simulink library "FadeControlBtc"  (R2022b)
settings: Solver=VariableStepAuto  StartTime=0.0  StopTime=10.0  RelTol=1e-3
undefined symbols (not defined in the file or in its folder): Row
libraries: TuneVar x6, TOP x2, FeaturePath x1, HandyTextFile x1, RTC x1
settings Model: Creator=kl13806  LastModifiedBy=kl13806
settings SolverCC: AlgebraicLoopSolver=TrustRegion
settings DebuggingCC: UnconnectedInputMsg=warning  UnconnectedOutputMsg=warning  UnconnectedLineMsg=warning  SFMachineParentedDataDiag=warning
settings ModelReferenceCC: EnableRefExpFcnMdlSchedulingChecks=on
settings RTWCC: DLArmComputeVersion=19.05

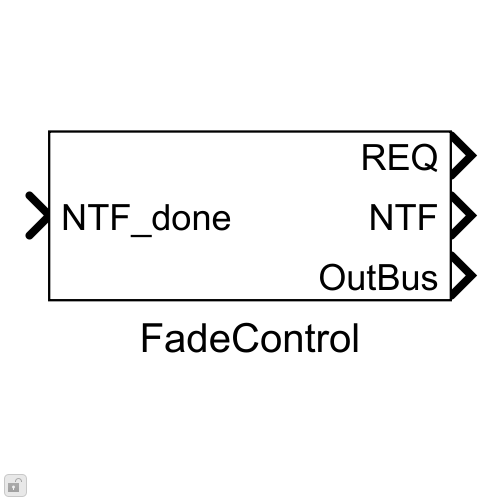
[thumbnail: Simulink's stored preview of the top-level diagram]
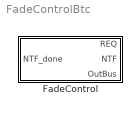
== system FadeControlBtc ==
  FadeControl : Subsystem  mask(Blocklib FadeControl){Config=[], FeatureName=FadeControl}
      mask prompts: Config "FadeControlConfig"; FeatureName "Feature path name:"
      mask help: This component is to be used in conjunction with 1 or more instances of the FadeRamper block. It provides the control layer for Fade processing via an RTC and tune variables.
      mask init:
      | blkh=gcbh;
      | Config=BTConfig.Assert(blkh,Config);
      | Config.Validate();
      | BTConfig.InitSetFeatureIfPresent(blkh,'FeatureName');
      | 
      | % Set boundary conditions
      | rampRateBounds = [5,50000];
      | rampTimeBounds = [1,3000];
      mask Help: If this control block is being used in a "multi-instance" manner, i.e. it is contorlling two or more FadeRamper blocks, there is an additional step that must be done. The developer must add a function-triggered subsytem containing an AND logic gate, which will combine the notification completion signals of the multiple ramper instances. The output of this subsytem must then feed the NTF_done input of the FadeControl block.
      mask Callback Config: BTConfig.CallbackHideIfPresent(gcbh,{'FeatureName'});
      mask TypeOptions FeatureName: FeaturePath/FeatureName

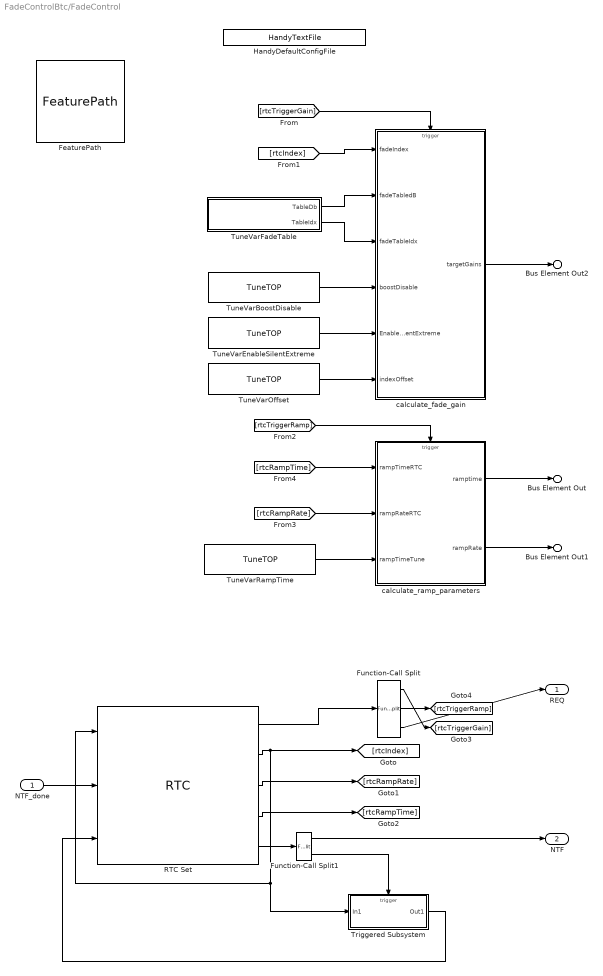
== system FadeControlBtc/FadeControl ==
  NTF_done : Inport
  FeaturePath : FeaturePath/FeaturePath  FeatureName=FadeControl  IsGroup=off  GroupNumber=-1  IsModule=off  TriggerInit=[320 214 435 321]
      settings: SourceProductName=Bose Talaria
  Function-Call Split : FunctionCallSplit  IconShape=distinctive  NumOutputPorts=3
  Function-Call Split1 : FunctionCallSplit  IconShape=distinctive  NumOutputPorts=2  OutputPortLayout=default
  HandyDefaultConfigFile : HandyTextFile/HandyTextFile  TemplateSource=Config  FileSuffix=Init  OpenDialogOnLoad=off  UseThisBlockName=off  AddGrandParentNamePrefix=off  TheDefaultText=|  ShowInLibBrowser=on
      | % $(FILENAME) Setup model parameters for each "Init" callback (e.g. update diagram)
      | sample_rate_in_hertz = 44100;
      | frame_size = 32;
      | sysin_channel_count = 2;
      settings: SourceProductName=Bose Talaria
  RTC Set : RTC/RTC  Description=|  REQ_Priority=RTC_Mask.NormalPriority  RequestAtInit=off  EnableRequest=on  REQElemName1=gain_index  REQElemType1=uint32  REQElemWidth1=1  REQElemInitial1=[]  REQElemName2=ramp_db_per_second  REQElemType2=uint32  REQElemWidth2=1  REQElemInitial2=[]  REQElemName3=ramp_milliseconds  REQElemType3=uint32  REQElemWidth3=1  REQElemInitial3=[]  REQElemType4=uint32  REQElemWidth4=1  REQElemInitial4=[]  REQElemType5=uint32  REQElemWidth5=1  REQElemInitial5=[]  REQElemType6=uint32  REQElemWidth6=1  REQElemInitial6=[]  REQElemType7=uint32  REQElemWidth7=1  REQElemInitial7=[]  REQElemType8=uint32  REQElemWidth8=1  REQElemInitial8=[]  REQElemType9=uint32  REQElemWidth9=1  REQElemInitial9=[]  REQElemType10=uint32  REQElemWidth10=1  REQElemInitial10=[]  EnableResponse=on  EnableRSP_StatusIn=off  RSPElemName1=gain_index  RSPElemType1=uint32  RSPElemWidth1=1  RSPElemType2=uint32  RSPElemWidth2=1  RSPElemType3=uint32  RSPElemWidth3=1  RSPElemType4=uint32  RSPElemWidth4=1  RSPElemType5=uint32  RSPElemWidth5=1  RSPElemType6=uint32  RSPElemWidth6=1  RSPElemType7=uint32  RSPElemWidth7=1  RSPElemType8=uint32  RSPElemWidth8=1  RSPElemType9=uint32  RSPElemWidth9=1  RSPElemType10=uint32  RSPElemWidth10=1  EnableNotification=on  EnableNTF_PrepTrig=off  NTFElemName1=gain_index  NTFElemType1=uint32  NTFElemWidth1=1  NTFElemType2=uint32  NTFElemWidth2=1  NTFElemType3=uint32  NTFElemWidth3=1  NTFElemType4=uint32  NTFElemWidth4=1  NTFElemType5=uint32  NTFElemWidth5=1  NTFElemType6=uint32  NTFElemWidth6=1  NTFElemType7=uint32  NTFElemWidth7=1  NTFElemType8=uint32  NTFElemWidth8=1  NTFElemType9=uint32  NTFElemWidth9=1  NTFElemType10=uint32  NTFElemWidth10=1  MaskMessageName=Set
      | Provide the target value as a 32-bit signed integer index value (to be mapped through a tunable calibration into a normalized float between -1 and 1).
      |  
      | To use slope-based ramping:
      | ----------------------------------
      | When db_per_second has a non-zero value,ramp_milliseconds is ignored and db_per_second controls the ramp.
      |  
      | To use time-based ramping:
      | ----------------------------------
      | The value of db_per_second must be zero for ramp milliseconds to then control the ramping.
      settings: SourceProductName=Bose Talaria
  Triggered Subsystem : Subsystem  TreatAsAtomicUnit=on
  TuneVarBoostDisable : TuneVar/TuneTOP  Description=Specifies the the 'boost' value to be applied to the channels towards which the fade is shifted. A value of '1' indicates that there is no boost (i.e. 0 dB), whereas '0' indicates that the 'boost' must be computed from the 'cut' value (which gets computed from the Table). In order to preserve the overall energy, the following formula is used: Boost^2 + Cut^2 = 2.  TriggerInit=[545 540 690 580]  TopName=BoostDisable  TuneName=BoostDisable  DataType=single  TunabilityNumber=2  MinValue=[]  MaxValue=[]  BankNumber=Config.BankNumber  PreOverlay=false  PostOverlay=false  UseSameName=on  MaskValue=Config.DefaultBoostDisable
      settings: SourceProductName=Bose Talaria
  TuneVarEnableSilentExtreme : TuneVar/TuneTOP  Description=|  TriggerInit=[545 600 690 640]  TopName=EnableSilentExtreme  TuneName=EnableSilentExtreme  DataType=single  TunabilityNumber=2  MinValue=[]  MaxValue=[]  BankNumber=Config.BankNumber  PreOverlay=false  PostOverlay=false  UseSameName=on  MaskValue=Config.DefaultSilentExtreme
      | When set to '0', the fade process occurs as follows- Only the non-bass content of the audio is faded and the bass content of the corresponding group remains as it is. This means that at extreme indices, the bass content of the group whose audio received a gain 'cut' is still intact.
      | 
      | When set to '1', if the audio is faded *completely* forward or backward (extreme indices), the group which is faded out is muted (both bass and non-bass content).
      settings: SourceProductName=Bose Talaria
  TuneVarFadeTable : Subsystem  Description=Map indices to corresponding gains in dB. Gains for indices located between consecutive index entries in the table are computed linearly.
  TuneVarOffset : TuneVar/TuneTOP  Description=Defines the index at which the Fade is at the center.  TriggerInit=[545 660 690 700]  TopName=offset  TuneName=offset  DataType=single  TunabilityNumber=2  MinValue=[]  MaxValue=[]  BankNumber=Config.BankNumber  PreOverlay=false  PostOverlay=false  UseSameName=on  MaskValue=Config.DefaultIndexOffset
      settings: SourceProductName=Bose Talaria
  TuneVarRampTime : TuneVar/TuneTOP  Description=Specifies the default ramp time for the rampers.  TriggerInit=[540 845 685 885]  TopName=RampTime  TuneName=RampTime  DataType=single  TunabilityNumber=2  MinValue=[]  MaxValue=[]  BankNumber=0  PreOverlay=false  PostOverlay=false  UseSameName=on  MaskValue=Config.DefaultRampTimeMs
      settings: SourceProductName=Bose Talaria
  calculate_fade_gain : MATLAB Function  TreatAsAtomicUnit=on  mask{MaskNumRampers=Config.NumRampers}
  calculate_ramp_parameters : MATLAB Function  TreatAsAtomicUnit=on
  REQ : Outport
  NTF : Outport  Port=2
  Bus Element Out : Outport  Port=3  PortName=OutBus  Element=rampTimeMs
  Bus Element Out1 : Outport  Port=3  PortName=OutBus  Element=rampRateDbPerSecond
  Bus Element Out2 : Outport  Port=3  PortName=OutBus  Element=targetGains
  wires:
  Triggered Subsystem/1(Out1) -> RTC Set/3
  Function-Call Split1/2 -> Triggered Subsystem/Trigger
  Function-Call Split1/1 -> NTF/1
  RTC Set/5 -> Function-Call Split1/1
  RTC Set/1 -> Function-Call Split/1
  RTC Set/2 -> [rtcIndex], Triggered Subsystem/1(In1), RTC Set/1
  Function-Call Split/1 -> [rtcTriggerGain]
  Function-Call Split/3 -> REQ/1
  TuneVarOffset/1 -> calculate_fade_gain/6(indexOffset)
  TuneVarBoostDisable/1 -> calculate_fade_gain/4(boostDisable)
  TuneVarEnableSilentExtreme/1 -> calculate_fade_gain/5(EnableSilentExtreme)
  TuneVarFadeTable/1(TableDb) -> calculate_fade_gain/2(fadeTabledB)
  RTC Set/3 -> [rtcRampRate]
  RTC Set/4 -> [rtcRampTime]
  [rtcTriggerGain] -> calculate_fade_gain/Trigger
  [rtcIndex] -> calculate_fade_gain/1(fadeIndex)
  Function-Call Split/2 -> [rtcTriggerRamp]
  [rtcTriggerRamp] -> calculate_ramp_parameters/Trigger
  [rtcRampRate] -> calculate_ramp_parameters/2(rampRateRTC)
  [rtcRampTime] -> calculate_ramp_parameters/1(rampTimeRTC)
  TuneVarRampTime/1 -> calculate_ramp_parameters/3(rampTimeTune)
  calculate_ramp_parameters/2(rampRate) -> Bus Element Out1/1
  calculate_ramp_parameters/1(ramptime) -> Bus Element Out/1
  calculate_fade_gain/1(targetGains) -> Bus Element Out2/1
  TuneVarFadeTable/2(TableIdx) -> calculate_fade_gain/3(fadeTableIdx)
  NTF_done/1 -> RTC Set/2

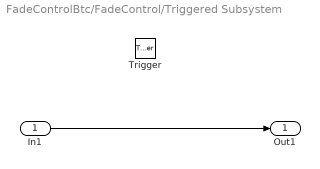
== system FadeControlBtc/FadeControl/Triggered Subsystem ==
  In1 : Inport
  Trigger : TriggerPort  TriggerType=function-call  VariantControl=Variant
  Out1 : Outport
  wires:
  In1/1 -> Out1/1

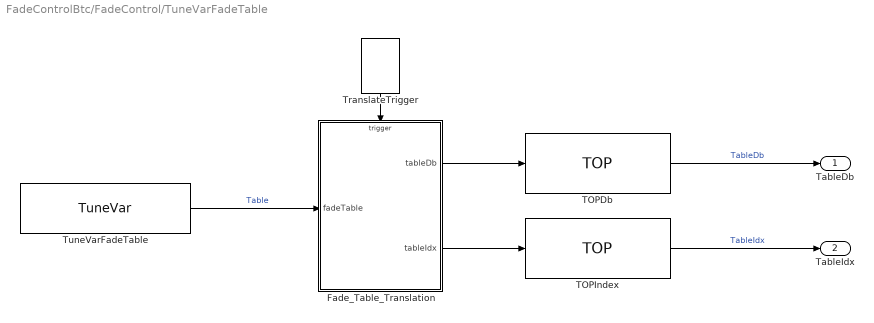
== system FadeControlBtc/FadeControl/TuneVarFadeTable ==
  Fade_Table_Translation : MATLAB Function  TreatAsAtomicUnit=on
  TOPDb : TOP/TOP  TriggerInit=[440 -5 585 55]  TopName=TableDb  DataType=single  BankNumber=Config.BankNumber  PreOverlay=false  PostOverlay=false  Role=Automatic
      settings: SourceProductName=Bose Talaria
  TOPIndex : TOP/TOP  TriggerInit=[440 80 585 140]  TopName=TableIdx  DataType=single  BankNumber=Config.BankNumber  PreOverlay=false  PostOverlay=false  Role=Automatic
      settings: SourceProductName=Bose Talaria
  TranslateTrigger : TuneVar/TranslateTrigger  TriggerInit=[276 -100 314 -45]
      settings: SourceProductName=Bose Talaria
  TuneVarFadeTable : TuneVar/TuneVar  Description=Define the fade curve using a table, with the first column being the list of indices and the second column being the corresponding fade gains in dB. Gain values for indices in between the elements in the table are linearly interpolated.  TuneName=Table  SpecifyMaxSize=on  VariableDim=1 (Row)  MaxSize=[30 2]  TunabilityNumber=3  MinValue=[]  MaxValue=[]  TriggerInit=[-65 45 105 95]  MaskValue=Config.DefaultIndex2DbTable
      settings: SourceProductName=Bose Talaria
  TableDb : Outport  VectorParamsAs1DForOutWhenUnconnected=off
  TableIdx : Outport  Port=2  VectorParamsAs1DForOutWhenUnconnected=off
  wires:
  Fade_Table_Translation/1(tableDb) -> TOPDb/1
  TuneVarFadeTable/1 -> Fade_Table_Translation/1(fadeTable)  "Table"
  TOPDb/1 -> TableDb/1  "TableDb"
  TranslateTrigger/1 -> Fade_Table_Translation/Trigger
  TOPIndex/1 -> TableIdx/1  "TableIdx"
  Fade_Table_Translation/2(tableIdx) -> TOPIndex/1

== matlab function FadeControlBtc/FadeControl/calculate_ramp_parameters ==
  data: rampTimeRTC input; rampRateRTC input; ramptime output; rampTimeTune input; rampRate output; rampRateBounds parameter; rampTimeBounds parameter
  events: trigger input FUNCTION_CALL_EVENT
function [ramptime, rampRate]  = calculate_ramp_parameters(rampTimeRTC, rampRateRTC,...
    rampTimeTune,...
    rampRateBounds, rampTimeBounds)  % parameters
% Function to calculate ramp parameters
% 

% Ramp time and rate are provided to the block through RTC messages. However 
% in case neither of them are provided, the block will use the default ramp 
% time given in the tune variables.

    ramptime = single(rampTimeTune);
    rampRate = single(0);

    if (rampRateRTC)
        rampRate = single(rampRateRTC);
        rampRate = max(rampRateBounds(1), rampRate);
        rampRate = min(rampRateBounds(2), rampRate);
    end
    if (rampTimeRTC)
        ramptime = single(rampTimeRTC);
    end
    ramptime = max(rampTimeBounds(1), ramptime);
    ramptime = min(rampTimeBounds(2), ramptime);
end

== matlab function FadeControlBtc/FadeControl/TuneVarFadeTable/Fade_Table_Translation ==
  data: tableDb output; fadeTable input; tableIdx output
  events: trigger input FUNCTION_CALL_EVENT
function [tableDb, tableIdx] = fcn(fadeTable)
%#codegen

% Set up the size and datatype of our TOP outputs:
maxTableSize = numel(fadeTable.Value) / 2;
idxType = 'uint8';
idxStorageType = 'uint32';
dbType = 'single';
tableIdx = zeros(1,maxTableSize,idxStorageType);
tableDb = zeros(1,maxTableSize,dbType);

% separate the pairs into their index and value components
givenPairs = fadeTable.Size(1);
indexes = fadeTable.Value(1:givenPairs,1);
values = fadeTable.Value(1:givenPairs,2);

% then sort and ignore duplicates
[cleanIdx,map] = unique(indexes);

% Validate input sizes
numPairs = numel(map);
argName='FadeTable';

% Validate: enough data?
if (numPairs < 2)
    TranslateError('%s must have at least 2 index pairs. Encounted value with only %f pairs\n', argName, numPairs);
end

% Validate: Highest index still below 1.0?
if (cleanIdx(1) < 0 || cleanIdx(end) > intmax(idxType))
    TranslateError('%s out of range table index %f encountered. Index must be between 0 and 255.\n',argName,cleanIdx(end));
end

% fill in the table buffer with provided pairs
tableIdx(1:numPairs) = cleanIdx(1:numPairs);
tableDb(1:numPairs) = values(map(1:numPairs));

% fill the rest of the table buffer with the last entry
remainingPairs = numel(map)+1:maxTableSize;
tableIdx(remainingPairs) = tableIdx(numPairs);
tableDb(remainingPairs) =  tableDb(numPairs);

end

== matlab function FadeControlBtc/FadeControl/calculate_fade_gain ==
  data: fadeIndex input; fadeTabledB input; fadeTableIdx input; targetGains output size=[1,4]; boostDisable input; EnableSilentExtreme input; indexOffset input; MaskNumRampers parameter
  events: trigger input FUNCTION_CALL_EVENT
function targetGains  = Calculate_Fade_Gain(fadeIndex, fadeTabledB,...
    fadeTableIdx, boostDisable, EnableSilentExtreme, indexOffset, ... % inputs
    MaskNumRampers) % parameters

% Computes the fade gains for the 'Front' and 'Rear' groups based on the
% index. Based on the position of the index in the table, either group 
% receives a gain 'cut' or 'boost' in order to achieve the fade effect. The
% gain 'cut' is computed from the table and the 'boost' is in turn computed
% from the 'cut' value depending on whether 'boostDisable' is set (0dB) or
% reset. When reset, the boost value is computed from the cut value based 
% on the energy preseving relationship: Boost^2 + Cut^2 = 2. These gain 
% values are applied only to the non-bass frequencies; the bass remains 
% unaltered (unless 'silent extreme' is enabled). 

% Ramper configuration:
% 1 & 2: Non-bass (Front; Rear)
% 3 & 4: Bass (Front; Rear)

% global Rampers;
j = uint8(1);
cutLinearHighFreq = single(1.0);
cutLinearLowFreq = single(1.0);
targetGains = ones(1,MaskNumRampers,'single');
fadeIndex = single(fadeIndex);

% Find the front and the rear gains
% Based on the Fade table, the dB value of the index is calculated
while (j <= numel(fadeTableIdx))
    if (fadeIndex <= fadeTableIdx(j))
        if (j <= 1)  % First indexed value is linearly interpolated to zero
            if (fadeTableIdx(j))
                percent = single(fadeIndex) / single(fadeTableIdx(j));
            else
                percent = single(1);
            end
            cutLinearHighFreq = percent * 10 ^ (fadeTabledB(j) / 20);
        else         % Other values are interpolated in dB space
            lastIdx = fadeTableIdx(j-1);
            percent = single(fadeIndex - lastIdx) / single(fadeTableIdx(j) - lastIdx);
            cutLinearHighFreq = 10 ^ (((percent * (fadeTabledB(j) - fadeTabledB(j-1))) + fadeTabledB(j-1)) / 20);
        end
        break;
    else
        j = j + 1;
    end
end

% Compute boost gain
if boostDisable ~= 0
    boostLinearHighFreq = single(1);
else
    boostLinearHighFreq = sqrt(2.0 - cutLinearHighFreq^2);
end

% If silent extreme is enabled and we're extreme, make the cut complete
if (EnableSilentExtreme && abs(fadeIndex - indexOffset) >= (indexOffset-1))
    cutLinearHighFreq = single(0);
    cutLinearLowFreq = single(0);
end

% Assign to Gain Values
if (fadeIndex - indexOffset) < 0 % Front speakers attenuated
    targetGains(1) = single(cutLinearHighFreq);
    targetGains(2) = single(boostLinearHighFreq);
    targetGains(3) = single(cutLinearLowFreq);
    targetGains(4) = single(1.0);
else
    targetGains(1) = single(boostLinearHighFreq);
    targetGains(2) = single(cutLinearHighFreq);
    targetGains(3) = single(1.0);
    targetGains(4) = single(cutLinearLowFreq);
end
